simulink model "ASML_Plant"  (R2022a)
settings: Solver=FixedStepAuto  StartTime=0.0  StopTime=1  RelTol=1e-3
model workspace (MAT data in the model file):
  EnableFastRf = 1
  meanEuv = 5.86107747608
  rfPoly = Simulink.Parameter
  rfPoly.Value = [0 0.4 0.6]
  rfPoly.DataType = 'double'
  rfPoly.Complexity = 'real'
  rfPoly.Dimensions = [1 3]
values from neighbouring files (symbols this model uses):
  fastA = [0.843499158894  -0.0734778605106  -0.451310431629; 0.0734778605106  0.970278054134  0.0727505606866; 0  0  0]    [modelParams.mat]
  fastB = [0 0 1]    [modelParams.mat]
  fastC = [-0.451310431629 -0.0727505606866 0]    [modelParams.mat]
  fastD = 0    [modelParams.mat]
  InitRf = 0.627718676731    [modelParams.mat]
  rfPoly = [-0.05 0.35 0.7]    [modelParams.mat]
  skipDelayInt = 1    [modelParams.mat]
  slowA = 0.999997000004    [modelParams.mat]
  slowB = 1    [modelParams.mat]
  slowC = 0    [modelParams.mat]
  slowD = 1    [modelParams.mat]
  Ts = 20e-6    (= 2e-05)    [computeDose1Burst.m]    (also in computeDose1Burst_filtered.m; modelParams.mat)
libraries: simulink x2
settings Model: Creator=rjacques  LastModifiedBy=maxcr
settings SolverCC: AlgebraicLoopSolver=TrustRegion
settings DataIOCC: ReturnWorkspaceOutputs=off
settings DebuggingCC: UnconnectedInputMsg=warning  UnconnectedOutputMsg=warning  UnconnectedLineMsg=warning  SFMachineParentedDataDiag=warning  ArithmeticOperatorsInVariantConditions=warning
settings SFSimCC: SimUseLocalCustomCode=off  CustomCodeUndefinedFunction=UseInterfaceOnly
settings RTWCC: RTWUseLocalCustomCode=off  DLArmComputeVersion=19.05
settings CodeAppCC: StateflowObjectComments=on

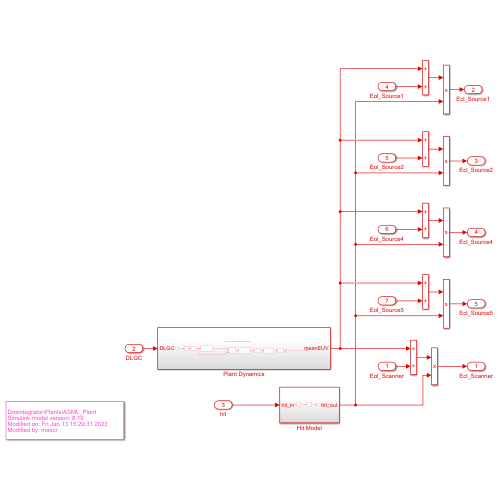
[thumbnail: Simulink's stored preview of the top-level diagram]
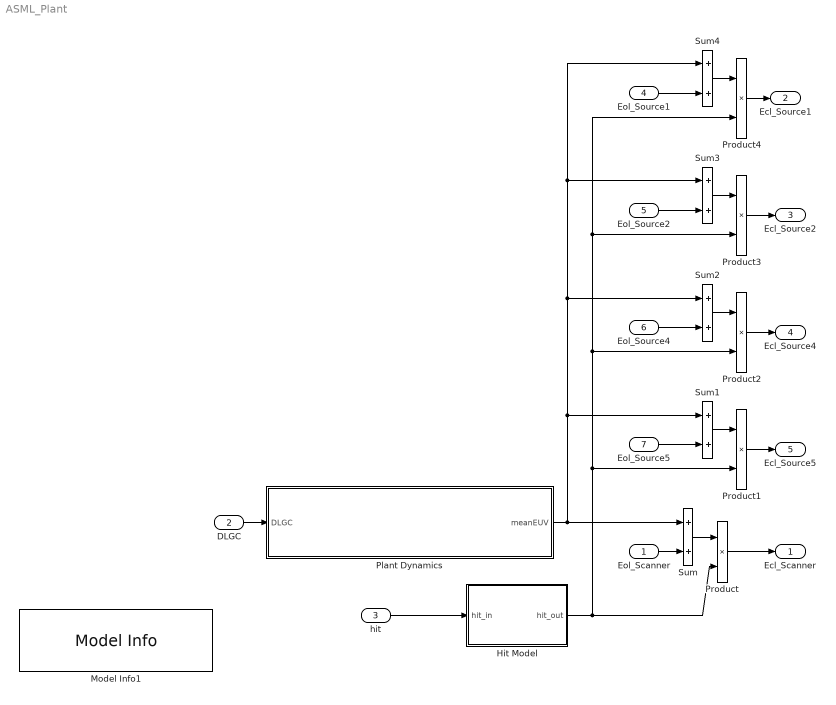
== system ASML_Plant ==
  Eol_Scanner : Inport  Unit=mJ  PortDimensions=1
  DLGC : Inport  Port=2  OutMin=0  OutMax=1  Unit=1  PortDimensions=1
  hit : Inport  Port=3  Unit=mJ  PortDimensions=1
  Eol_Source1 : Inport  Port=4  Unit=mJ  PortDimensions=1
  Eol_Source2 : Inport  Port=5  Unit=mJ  PortDimensions=1
  Eol_Source4 : Inport  Port=6  Unit=mJ  PortDimensions=1
  Eol_Source5 : Inport  Port=7  Unit=mJ  PortDimensions=1
  Hit Model : Subsystem
  Model Info1 : simulink/Model-Wide Utilities/Model Info  Frame=on  DisplayStringWithTags=|  HorizontalTextAlignment=Left  LeftAlignmentValue=0.02
      | Dosintegrator\Plants\%<ModelName>
      | Simulink model version: %<ModelVersion>
      | Modified on: %<LastModificationDate>
      | Modified by: %<ModifiedBy>
  Plant Dynamics : Subsystem
  Product{,1..4} (5 alike) : Product
  Sum{,1..4} (5 alike) : Sum
  Ecl_Scanner : Outport  Unit=mJ  VectorParamsAs1DForOutWhenUnconnected=off
  Ecl_Source1 : Outport  Port=2  Unit=mJ  VectorParamsAs1DForOutWhenUnconnected=off
  Ecl_Source2 : Outport  Port=3  Unit=mJ  VectorParamsAs1DForOutWhenUnconnected=off
  Ecl_Source4 : Outport  Port=4  Unit=mJ  VectorParamsAs1DForOutWhenUnconnected=off
  Ecl_Source5 : Outport  Port=5  Unit=mJ  VectorParamsAs1DForOutWhenUnconnected=off
  wires:
  Eol_Scanner/1 -> Sum/2
  Product/1 -> Ecl_Scanner/1
  Sum/1 -> Product/1
  DLGC/1 -> Plant Dynamics/1(DLGC)
  hit/1 -> Hit Model/1(hit_in)
  Hit Model/1(hit_out) -> Product2/2, Product4/2, Product3/2, Product1/2, Product/2
  Sum1/1 -> Product1/1
  Eol_Source5/1 -> Sum1/2
  Product1/1 -> Ecl_Source5/1
  Sum2/1 -> Product2/1
  Sum3/1 -> Product3/1
  Sum4/1 -> Product4/1
  Product4/1 -> Ecl_Source1/1
  Product3/1 -> Ecl_Source2/1
  Product2/1 -> Ecl_Source4/1
  Eol_Source4/1 -> Sum2/2
  Eol_Source2/1 -> Sum3/2
  Eol_Source1/1 -> Sum4/2
  Plant Dynamics/1(meanEUV) -> Sum2/1, Sum3/1, Sum4/1, Sum1/1, Sum/1

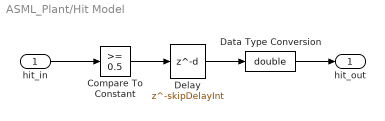
== system ASML_Plant/Hit Model ==
  hit_in : Inport  Unit=mJ  PortDimensions=1
  Compare To Constant : simulink/Logic and Bit Operations/Compare To Constant  relop=>=  const=0.5  OutDataTypeStr=boolean
  Data Type Conversion : DataTypeConversion  OutDataTypeStr=double  SaturateOnIntegerOverflow=off  RndMeth=Floor
  Delay : Delay  DelayLength=skipDelayInt  InitialCondition=1
  hit_out : Outport
  wires:
  Delay/1 -> Data Type Conversion/1
  hit_in/1 -> Compare To Constant/1
  Data Type Conversion/1 -> hit_out/1
  Compare To Constant/1 -> Delay/1

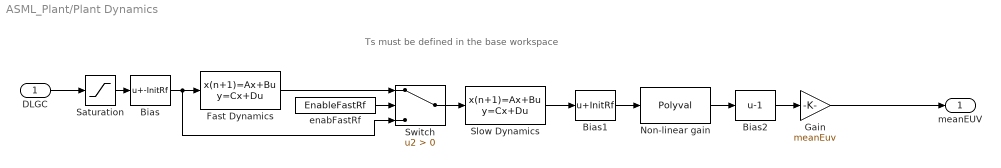
== system ASML_Plant/Plant Dynamics ==
  note: Ts must be defined in the base workspace
  DLGC : Inport
  Bias : Bias  Bias=-InitRf  SaturateOnIntegerOverflow=off
  Bias1 : Bias  Bias=InitRf  SaturateOnIntegerOverflow=off
  Bias2 : Bias  Bias=-1  SaturateOnIntegerOverflow=off
  Fast Dynamics : DiscreteStateSpace  A=fastA  B=fastB  C=fastC  D=fastD  SampleTime=Ts
  Gain : Gain  Gain=meanEuv
      settings: AttributesFormatString=%<Gain>
  Non-linear gain : Polyval  Coefs=rfPoly
      settings: AttributesFormatString=%<Description>
  Saturation : Saturate  Description=|  UpperLimit=1  LowerLimit=-inf
      | Limit the DLGC 
      | input to the range 
      | [0,1]
      settings: AttributesFormatString=%<Description>
  Slow Dynamics : DiscreteStateSpace  A=slowA  B=slowB  C=slowC  D=slowD  SampleTime=Ts
  Switch : Switch  Criteria=u2 > Threshold  SaturateOnIntegerOverflow=off  InputSameDT=off
  enabFastRf : Constant  Value=EnableFastRf
  meanEUV : Outport
  wires:
  Fast Dynamics/1 -> Switch/1
  Slow Dynamics/1 -> Bias1/1
  Bias1/1 -> Non-linear gain/1
  enabFastRf/1 -> Switch/2
  Gain/1 -> meanEUV/1
  Switch/1 -> Slow Dynamics/1
  Saturation/1 -> Bias/1
  Non-linear gain/1 -> Bias2/1
  Bias2/1 -> Gain/1
  Bias/1 -> Switch/3, Fast Dynamics/1
  DLGC/1 -> Saturation/1
